simulink model "DC"  (R2023a)
settings: Solver=VariableStepAuto  StartTime=0.0  StopTime=0.75  RelTol=1e-3
libraries: spsMosfetLib x4, spsVoltageMeasurementLib x2, spsACVoltageSourceLib x1, spsCurrentMeasurementLib x1, spsDCMachineLib x1, spsDCVoltageSourceLib x1, sps_lib x1
settings Model: Creator=vande  LastModifiedBy=vande

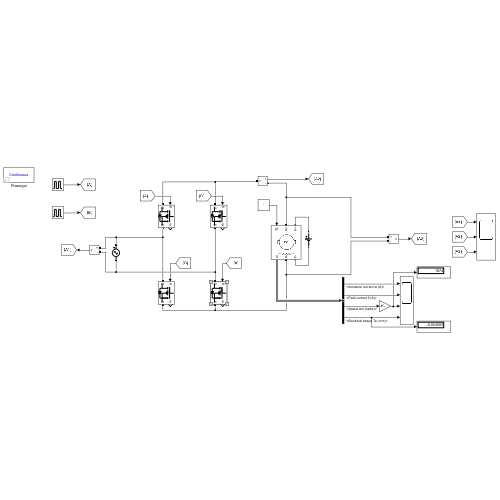
[thumbnail: Simulink's stored preview of the top-level diagram]
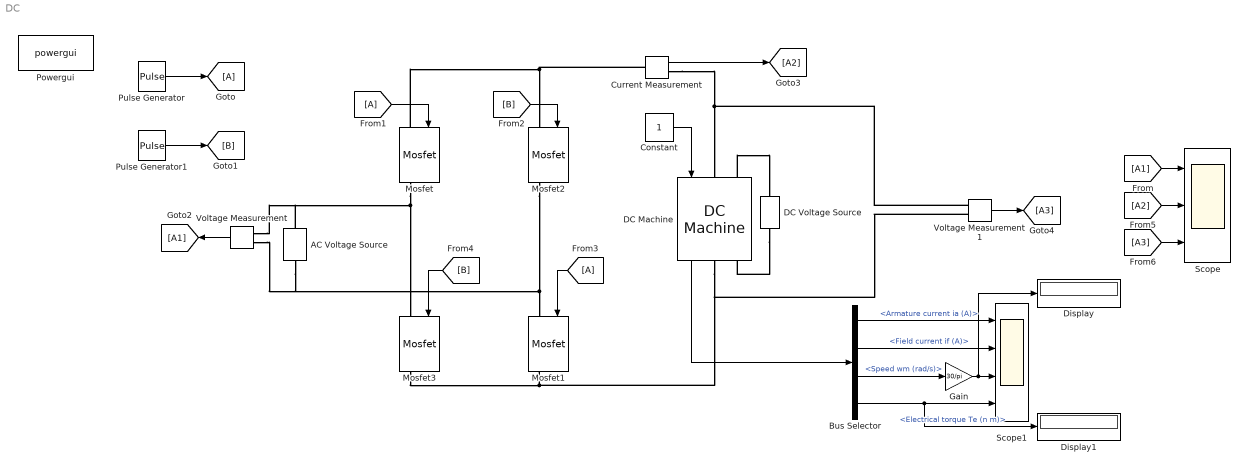
== system DC ==
  AC Voltage Source : spsACVoltageSourceLib/AC Voltage Source  Amplitude=339  Phase=0  Frequency=50  SampleTime=0  Measurements=None  BusType=swing  Pref=10e3  Qref=0  Qmin=-inf  Qmax=+inf
  Bus Selector : BusSelector  OutputSignals=Armature current ia (A),Field current if (A),Speed wm (rad/s),Electrical torque Te (n m)
  Constant : Constant
  Current Measurement : spsCurrentMeasurementLib/Current Measurement  PhasorSimulation=off  OutputType=Complex  PSBequivalent=0
  DC Machine : spsDCMachineLib/DC Machine  PresetModel=02: 5HP 240V 1750RPM Field:150V  MechanicalLoad=Torque TL  FieldType=Wound  ShowDetailedParameters=on  MeasurementBus=off  RLa=[0.78 0.016]  RLf=[150 112.5]  Laf=1.234  MachineConstant=Torque constant (N.m/A)  Ke=1.8  Kt=1.8  J=0.05  Bm=0.01  Tf=0  w0=1  Ifinit=1  TsPowergui=0  TsBlock=-1
  DC Voltage Source : spsDCVoltageSourceLib/DC Voltage Source  Amplitude=150  Measurements=None
  Display : Display
  Display1 : Display
  From1 : From
  From3 : From
  Gain : Gain  Gain=30/pi
  Goto : Goto
  Mosfet{,1..3} (4 alike) : spsMosfetLib/Mosfet  Ron=0.1  Lon=0  Rd=0.01  Vfd=0  IC=0  Rs=1e5  Cs=inf  Measurements=on
  Powergui : sps_lib/powergui  Priority=1  SimulationMode=Continuous  SampleTime=50e-6  frequency=60  Iterations=50  frequencyindice=50  Pbase=100e6  ErrMax=1e-4  UnitsV=kV  UnitsW=MW  buscounter=0  FunctionMessages=off  echomessages=off  EnableUseOfTLC=off  CurrentSourceSwitches=off  DisableSnubberDevices=off  DisableRonSwitches=off  DisableVfSwitches=off  DisplayEquations=off  AutomaticDiscreteSolvers=off  SolverType=Tustin/Backward Euler (TBE)  Interpol=off  ExternalGateDelay=off  methode=off  Ts=100  x0status=blocks  SPID=on  SwTol=0  HookPort=off  NonlinearTolerance=1e-4  nMaxIteration=100  ContinueOnMaxIteration=off  RestoreLinks=warning  ResistiveCurrentMeasurement=off  Frange=[0:2:500]  Ylog=off  Xlog=on  ShowGrid=off  save=off  variable=ZData  structure=0  ZoomFFT=off  StartTime=0.0  cycles=1  DisplayStyle=1  fundamental=60  FreqAxis=off  MaxFrequency=1000  frequencyindicesteady=1  RmsSteady=1  display=off
  Pulse Generator : DiscretePulseGenerator  PulseType=Time based  Period=10  PulseWidth=5
  Pulse Generator1 : DiscretePulseGenerator  PulseType=Time based  Period=10  PulseWidth=5  PhaseDelay=5
  Scope : Scope  NumInputPorts=3
  Scope1 : Scope  NumInputPorts=4
  Voltage Measurement : spsVoltageMeasurementLib/Voltage Measurement  PhasorSimulation=off  OutputType=Complex  PSBequivalent=0
  Voltage Measurement1 : spsVoltageMeasurementLib/Voltage Measurement  PhasorSimulation=off  OutputType=Complex  PSBequivalent=0
  wires:
  [A1] -> Scope/1
  Pulse Generator/1 -> Goto/1
  Pulse Generator1/1 -> [B]
  From1/1 -> Mosfet/1
  From3/1 -> Mosfet1/1
  [B] -> Mosfet2/1
  [B] -> Mosfet3/1
  Constant/1 -> DC Machine/1
  DC Machine/1 -> Bus Selector/1
  Current Measurement/1 -> [A2]
  Voltage Measurement/1 -> [A1]
  Voltage Measurement1/1 -> [A3]
  [A2] -> Scope/2
  [A3] -> Scope/3
  Bus Selector/1 -> Scope1/1  "<Armature current ia (A)>"
  Bus Selector/2 -> Scope1/2  "<Field current if (A)>"
  Bus Selector/3 -> Gain/1  "<Speed wm (rad/s)>"
  Bus Selector/4 -> Display1/1, Scope1/4  "<Electrical torque Te (n m)>"
  Gain/1 -> Display/1, Scope1/3
  connections:
  Mosfet/RConn1 -- Voltage Measurement/LConn1 -- AC Voltage Source/RConn1 -- Mosfet3/LConn1
  Mosfet2/RConn1 -- AC Voltage Source/LConn1 -- Voltage Measurement/LConn2 -- Mosfet1/LConn1
  DC Machine/LConn2 -- DC Voltage Source/RConn1
  DC Voltage Source/LConn1 -- DC Machine/RConn2
  Current Measurement/RConn1 -- Voltage Measurement1/LConn1 -- DC Machine/LConn1
  Mosfet/LConn1 -- Current Measurement/LConn1 -- Mosfet2/LConn1
  Mosfet3/RConn1 -- Voltage Measurement1/LConn2 -- DC Machine/RConn1 -- Mosfet1/RConn1
